simulink model "test_9x8_strobe"  (Simulink 7.4)
settings: Solver=ode45  StartTime=0  StopTime=1000  RelTol=1e-3
libraries: xbsIndex_r4 x19, isi_correlator_lib x1
settings Model: Creator=wjm  LastModifiedBy=wjm

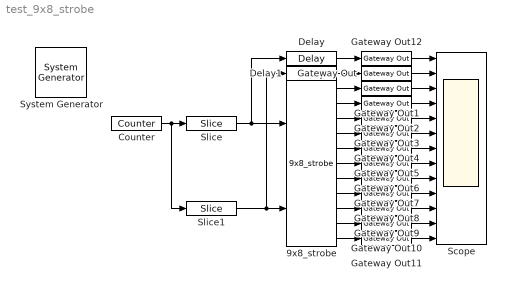
== system test_9x8_strobe ==
  " System Generator" : xbsIndex_r4/ System Generator  Tag=genX  SystemSampleTime=-1  xilinxfamily=Virtex6  part=xc6vsx315t  speed=-3  package=ff1156  synthesis_tool=XST  clock_wrapper=Clock Enables  directory=./netlist  testbench=off  simulink_period=1  sysclk_period=10  dcm_input_clock_period=10  incr_netlist=off  trim_vbits=Everywhere in SubSystem  dbl_ovrd=According to Block Masks  core_generation=According to Block Masks  run_coregen=off  deprecated_control=off  eval_field=0  block_type=sysgen
      settings: block_version=11.3
  9x8_strobe : isi_correlator_lib/9x8_strobe  SystemSampleTime=-1
  Counter : xbsIndex_r4/Counter  cnt_type=Free Running  cnt_to=Inf  operation=Up  start_count=0  cnt_by_val=1  arith_type=Unsigned  n_bits=10  bin_pt=0  load_pin=off  rst=off  en=off  explicit_period=on  period=1  dbl_ovrd=off  use_behavioral_HDL=off  implementation=Fabric  block_type=counter
      settings: block_version=11.3
  Delay : xbsIndex_r4/Delay  en=off  latency=2  dbl_ovrd=off  reg_retiming=on  block_type=delay
      settings: block_version=11.3
  Delay1 : xbsIndex_r4/Delay  en=off  latency=2  dbl_ovrd=off  reg_retiming=on  block_type=delay
      settings: block_version=11.3
  Gateway Out{,1..12} (13 alike) : xbsIndex_r4/Gateway Out  hdl_port=on  timing_constraint=None  locs_specified=off  LOCs={}  block_type=gatewayout
      settings: infoedit="Gateway out block.  Converts Xilinx fixed point inputs into ouputs of type Simulink integer, double, or fixed point.<br><br>Hardware notes:  In hardware these blocks become top level output ports or are discarded, depending on how they are configured."  block_version=11.3
  Scope : Scope  NumInputPorts=13
      settings: YMin=-5~-5~-5~-5~-5~-5~-5~-5~-5~-5~-5~-5~-5  YMax=5~5~5~5~5~5~5~5~5~5~5~5~5
  Slice : xbsIndex_r4/Slice  nbits=1  boolean_output=on  mode=Lower Bit Location + Width  bit1=0  base1=MSB of Input  bit0=6  base0=LSB of Input  dbl_ovrd=off  block_type=slice
      settings: block_version=11.3
  Slice1 : xbsIndex_r4/Slice  nbits=1  boolean_output=on  mode=Lower Bit Location + Width  bit1=0  base1=MSB of Input  bit0=9  base0=LSB of Input  dbl_ovrd=off  block_type=slice
      settings: block_version=11.3
  wires:
  Counter/1 -> Slice/1, Slice1/1
  9x8_strobe/1 -> Gateway Out1/1
  9x8_strobe/2 -> Gateway Out2/1
  9x8_strobe/3 -> Gateway Out3/1
  9x8_strobe/4 -> Gateway Out4/1
  9x8_strobe/5 -> Gateway Out5/1
  9x8_strobe/6 -> Gateway Out6/1
  9x8_strobe/7 -> Gateway Out7/1
  9x8_strobe/8 -> Gateway Out8/1
  9x8_strobe/9 -> Gateway Out9/1
  9x8_strobe/10 -> Gateway Out10/1
  9x8_strobe/11 -> Gateway Out11/1
  Slice/1 -> 9x8_strobe/1, Delay/1
  Gateway Out12/1 -> Scope/1
  Gateway Out/1 -> Scope/2
  Gateway Out1/1 -> Scope/3
  Gateway Out2/1 -> Scope/4
  Gateway Out3/1 -> Scope/5
  Gateway Out4/1 -> Scope/6
  Gateway Out5/1 -> Scope/7
  Gateway Out6/1 -> Scope/8
  Gateway Out7/1 -> Scope/9
  Gateway Out8/1 -> Scope/10
  Gateway Out9/1 -> Scope/11
  Gateway Out10/1 -> Scope/12
  Gateway Out11/1 -> Scope/13
  Delay/1 -> Gateway Out12/1
  Delay1/1 -> Gateway Out/1
  Slice1/1 -> 9x8_strobe/2, Delay1/1
